simulink model "sampleModel111"  (Simulink 9.1)
settings: Solver=VariableStepAuto  StartTime=0.0  StopTime=10.0  RelTol=1e-3
undefined symbols (not defined in the file): DiscIntNeverNeededParam, Newton, Raphson
libraries: simulink x41
(part 1 of 2)
settings Model: Creator=DELL  LastModifiedBy=DELL
settings DataIOCC: SaveFormat=Dataset
settings OptimizationCC: LifeSpan=auto
settings DebuggingCC: UnderspecifiedInitializationDetection=Simplified  MergeDetectMultiDrivingBlocksExec=error  SFUnexpectedBacktrackingDiag=error  SFNoUnconditionalDefaultTransitionDiag=error  SFExecutionAtInitializationDiag=warning
settings HardwareCC: ProdBitPerPointer=64  ProdBitPerSizeT=64  ProdBitPerPtrDiffT=64  ProdLargestAtomicFloat=Float  ProdIntDivRoundTo=Zero  ProdEndianess=LittleEndian  ProdWordSize=64  ProdHWDeviceType=Intel->x86-64 (Windows64)
settings ModelReferenceCC: PropagateSignalLabelsOutOfModel=on
settings CodeAppCC: StateflowObjectComments=off
settings GRTTargetCC: TargetLangStandard=C99 (ISO)  CombineOutputUpdateFcns=on  GRTInterface=off
settings ConfigComp: CovMetricSettings=dwe  CovHtmlReporting=off  CovSaveCumulativeToWorkspaceVar=off  CovSaveSingleToWorkspaceVar=off  CovExternalEMLEnable=on

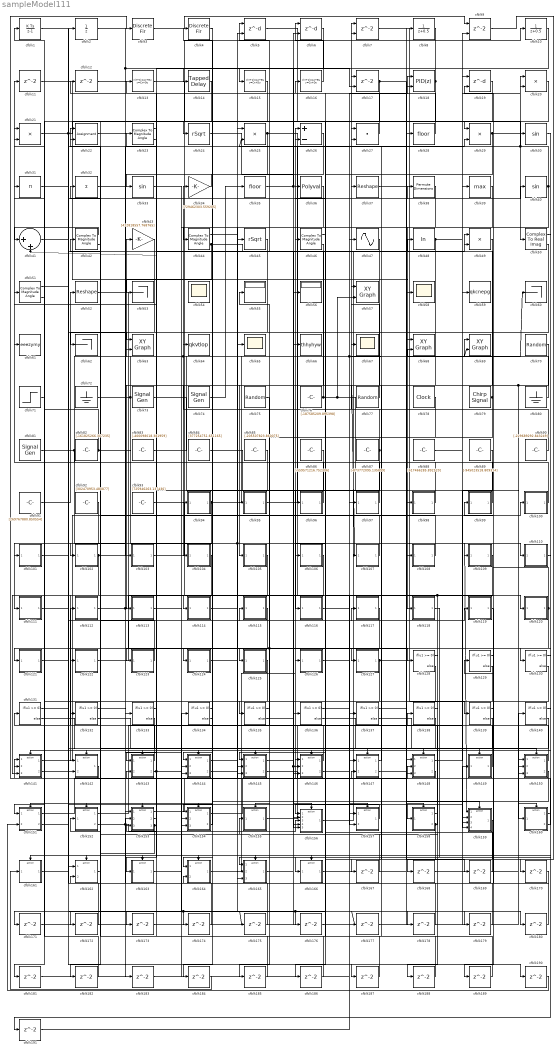
== system sampleModel111 ==
  cfblk1 : DiscreteIntegrator  ICPrevOutput=DiscIntNeverNeededParam  ICPrevScaledInput=DiscIntNeverNeededParam
  cfblk10 : DiscreteTransferFcn  SampleTime=1
  cfblk100 : Subsystem
  cfblk101 : Subsystem
  cfblk102 : Subsystem
  cfblk103 : Subsystem
  cfblk104 : Subsystem
  cfblk105 : Subsystem
  cfblk106 : Subsystem
  cfblk107 : Subsystem
  cfblk108 : Subsystem
  cfblk109 : Subsystem
  cfblk{11..12,167..191} (27 alike) : Delay  SampleTime=1
  cfblk110 : Subsystem
  cfblk111 : Subsystem
  cfblk112 : Subsystem
  cfblk113 : Subsystem
  cfblk114 : Subsystem
  cfblk115 : Subsystem
  cfblk116 : Subsystem
  cfblk117 : Subsystem
  cfblk118 : Subsystem
  cfblk119 : Subsystem
  cfblk120 : Subsystem
  cfblk121 : Subsystem
  cfblk122 : Subsystem
  cfblk123 : Subsystem
  cfblk124 : Subsystem
  cfblk125 : Subsystem
  cfblk126 : Subsystem
  cfblk127 : Subsystem
  cfblk{128..140} (13 alike) : If  IfExpression=u1 >= 0  SampleTime=1
  cfblk13 : DiscreteStateSpace
  cfblk14 : simulink/Discrete/Tapped Delay  vinit=0.0  samptime=-1  NumDelays=1  DelayOrder=Oldest  includeCurrent=off
  cfblk141 : Subsystem  TreatAsAtomicUnit=on
  cfblk142 : Subsystem  TreatAsAtomicUnit=on
  cfblk143 : Subsystem  TreatAsAtomicUnit=on
  cfblk144 : Subsystem  TreatAsAtomicUnit=on
  cfblk145 : Subsystem  TreatAsAtomicUnit=on
  cfblk146 : Subsystem  TreatAsAtomicUnit=on
  cfblk147 : Subsystem  TreatAsAtomicUnit=on
  cfblk148 : Subsystem  TreatAsAtomicUnit=on
  cfblk149 : Subsystem  TreatAsAtomicUnit=on
  cfblk15 : DiscreteStateSpace
  cfblk150 : Subsystem  TreatAsAtomicUnit=on
  cfblk151 : Subsystem  TreatAsAtomicUnit=on
  cfblk152 : Subsystem  TreatAsAtomicUnit=on
  cfblk153 : Subsystem  TreatAsAtomicUnit=on
  cfblk154 : Subsystem  TreatAsAtomicUnit=on
  cfblk155 : Subsystem  TreatAsAtomicUnit=on
  cfblk156 : Subsystem  TreatAsAtomicUnit=on
  cfblk157 : Subsystem  TreatAsAtomicUnit=on
  cfblk158 : Subsystem  TreatAsAtomicUnit=on
  cfblk159 : Subsystem  TreatAsAtomicUnit=on
  cfblk16 : DiscreteStateSpace
  cfblk160 : Subsystem  TreatAsAtomicUnit=on
  cfblk161 : Subsystem  TreatAsAtomicUnit=on
  cfblk162 : Subsystem  TreatAsAtomicUnit=on
  cfblk163 : Subsystem  TreatAsAtomicUnit=on
  cfblk164 : Subsystem  TreatAsAtomicUnit=on
  cfblk165 : Subsystem  TreatAsAtomicUnit=on
  cfblk166 : Subsystem  TreatAsAtomicUnit=on
  cfblk17 : Delay  ShowEnablePort=on  SampleTime=1
      settings: InputPortMap=u0,e6
  cfblk18 : simulink/Continuous/PID Controller (2DOF)  Controller=PID  TimeDomain=Discrete-time  SampleTime=1  IntegratorMethod=Forward Euler  FilterMethod=Forward Euler  Form=Parallel  UseFilter=on  ControllerParametersSource=internal  P=1  I=1  D=0  N=100  b=1  c=1  InitialConditionSource=internal  InitialConditionForIntegrator=0  InitialConditionForFilter=0  ExternalReset=none  LimitOutput=off  UpperSaturationLimit=inf  LowerSaturationLimit=-inf  LinearizeAsGain=off  AntiWindupMode=none  Kb=1  TrackingMode=off  Kt=1  PParamMin=[]  PParamMax=[]  IParamMin=[]  IParamMax=[]  DParamMin=[]  DParamMax=[]  NParamMin=[]  NParamMax=[]  bParamMin=[]  bParamMax=[]  cParamMin=[]  cParamMax=[]  KbParamMin=[]  KbParamMax=[]  KtParamMin=[]  KtParamMax=[]  POutMin=[]  POutMax=[]  IOutMin=[]  IOutMax=[]  DOutMin=[]  DOutMax=[]  NOutMin=[]  NOutMax=[]  bOutMin=[]  bOutMax=[]  cOutMin=[]  cOutMax=[]  KbOutMin=[]  KbOutMax=[]  KtOutMin=[]  KtOutMax=[]  IntegratorOutMin=[]  IntegratorOutMax=[]  FilterOutMin=[]  FilterOutMax=[]  SumOutMin=[]  SumOutMax=[]  Sum1OutMin=[]  Sum1OutMax=[]  Sum2OutMin=[]  Sum2OutMax=[]  Sum3OutMin=[]  Sum3OutMax=[]  SumI1OutMin=[]  SumI1OutMax=[]  SumI2OutMin=[]  SumI2OutMax=[]  SumI3OutMin=[]  SumI3OutMax=[]  SumDOutMin=[]  SumDOutMax=[]  SaturationOutMin=[]  SaturationOutMax=[]  IntegratorContinuousStateAttributes=''  IntegratorStateMustResolveToSignalObject=off  IntegratorRTWStateStorageClass=Auto  FilterContinuousStateAttributes=''  FilterStateMustResolveToSignalObject=off  FilterRTWStateStorageClass=Auto  DifferentiatorICPrevScaledInput=0  DifferentiatorOutMin=[]  DifferentiatorOutMax=[]  FilterDiffOutCoefMin=[]  FilterDiffOutCoefMax=[]  SumDenOutMin=[]  SumDenOutMax=[]  SumNumOutMin=[]  SumNumOutMax=[]  ReciprocalOutMin=[]  ReciprocalOutMax=[]  DivideOutMin=[]  DivideOutMax=[]  TunerSelectOption=Transfer Function Based (PID Tuner App)
  cfblk19 : Delay  DelayLengthSource=Input port  SampleTime=1
      settings: InputPortMap=u0,p1
  cfblk2 : UnitDelay
  cfblk20 : Product  Inputs=**
  cfblk21 : Product  Inputs=**
  cfblk22 : Assignment  DiagnosticForDimensions=Warning  IndexOptions=Index vector (dialog)  Indices=1  OutputSizes=1
  cfblk{23,42,44,46,51} (5 alike) : ComplexToMagnitudeAngle
  cfblk24 : Sqrt  Operator=rSqrt  AlgorithmType=Newton-Raphson  SaturateOnIntegerOverflow=on
  cfblk25 : Product
  cfblk26 : Sum  Inputs=+-
  cfblk27 : DotProduct  InputSameDT=on  OutDataTypeStr=Inherit: Inherit via internal rule
  cfblk28 : Rounding
  cfblk29 : Product  Inputs=**
  cfblk3 : DiscreteFir  SampleTime=1
  cfblk30 : Trigonometry
  cfblk31 : Product  Inputs=*
  cfblk32 : Sum  Inputs=+
  cfblk33 : Trigonometry
  cfblk34 : Gain  Gain=[729462303.559205]
  cfblk35 : Rounding
  cfblk36 : Polyval  Coefs=[ +2.081618890e-019, -1.441693666e-014, +4.719686976e-010, -8.536869453e-006, +1.621573104e-001, -8.087801117e+001 ]
  cfblk37 : Reshape
  cfblk38 : PermuteDimensions
  cfblk39 : MinMax  Function=max
  cfblk4 : DiscreteFir  SampleTime=1
  cfblk40 : Trigonometry
  cfblk41 : Sum  Inputs=|++
  cfblk43 : Gain  Gain=[412818557.768765]
  cfblk45 : Sqrt  Operator=rSqrt  AlgorithmType=Newton-Raphson  SaturateOnIntegerOverflow=on
  cfblk47 : Sin  TimeSource=Use external signal  SampleTime=0
  cfblk48 : Math  Operator=log  SaturateOnIntegerOverflow=on
  cfblk49 : Product
  cfblk5 : Delay  DelayLengthSource=Input port  SampleTime=1
      settings: InputPortMap=u0,p1
  cfblk50 : ComplexToRealImag
  cfblk52 : Reshape
  cfblk53 : Terminator
  cfblk{54,58,65,67} (4 alike) : Scope
      cfblk54 settings: Floating=on
  cfblk55 : Display
  cfblk56 : Display
  cfblk{57,63,68..69} (4 alike) : simulink/Sinks/XY Graph  xmin=-1  xmax=1  ymin=-1  ymax=1  st=-1
  cfblk59 : ToWorkspace  VariableName=qkcnepg  SaveFormat=Timeseries  SampleTime=-1
  cfblk6 : Delay  DelayLengthSource=Input port  SampleTime=1
      settings: InputPortMap=u0,p1
  cfblk60 : Terminator
  cfblk61 : ToWorkspace  VariableName=eeezymy  SaveFormat=Timeseries  SampleTime=-1
  cfblk62 : Terminator
  cfblk64 : ToWorkspace  VariableName=qkvtlop  SaveFormat=Timeseries  SampleTime=-1
  cfblk66 : ToWorkspace  VariableName=thhyhyw  SaveFormat=Timeseries  SampleTime=-1
  cfblk7 : Delay  ShowEnablePort=on  SampleTime=1
      settings: InputPortMap=u0,e6
  cfblk70 : RandomNumber  Mean=[-93187.376150]  Variance=[1459.067159]  Seed=[649544594.000000]  SampleTime=0.1
  cfblk71 : Step  Time=[20.000000]  Before=[-473754726.003324]  After=[611327295.149890]  SampleTime=0
  cfblk72 : Ground
  cfblk73 : SignalGenerator  WaveForm=square  Amplitude=[306363798.887953]
  cfblk74 : SignalGenerator  WaveForm=square  Amplitude=[94323336.966715]
  cfblk75 : RandomNumber  Mean=[-15248.816156]  Variance=[85638.241331]  Seed=[321907178.000000]  SampleTime=0.1
  cfblk76 : Constant  Value=[-187585209.895398]  SampleTime=1
  cfblk77 : RandomNumber  Mean=[-59356.286087]  Variance=[90170.885384]  Seed=[654352613.000000]  SampleTime=0.1
  cfblk78 : DigitalClock
  cfblk79 : simulink/Sources/Chirp Signal  f1=[-120890436.083449]  T=[764356880.898604]  f2=[390283398.799809]
  cfblk8 : DiscreteTransferFcn  SampleTime=1
  cfblk80 : Ground
  cfblk81 : SignalGenerator  WaveForm=square  Amplitude=[-879054946.376527]  Units=rad/sec
  cfblk82 : Constant  Value=[-161825266.307235]  SampleTime=1
  cfblk83 : Constant  Value=[-400098018.381959]  SampleTime=1
  cfblk84 : Constant  Value=[377254751.651165]  SampleTime=1
  cfblk85 : Constant  Value=[-205507823.860075]  SampleTime=1
  cfblk86 : Constant  Value=[-559571216.752306]  SampleTime=1
  cfblk87 : Constant  Value=[-873772095.135899]  SampleTime=1
  cfblk88 : Constant  Value=[617466285.892520]  SampleTime=1
  cfblk89 : Constant  Value=[-945023518.809314]  SampleTime=1
  cfblk9 : Delay  ShowEnablePort=on  SampleTime=1
      settings: InputPortMap=u0,e6
  cfblk90 : Constant  Value=[-229689292.843249]  SampleTime=1
  cfblk91 : Constant  Value=[269767880.850554]  SampleTime=1
  cfblk92 : Constant  Value=[302470953.480877]  SampleTime=1
  cfblk93 : Constant  Value=[725946263.137430]  SampleTime=1
  cfblk94 : Subsystem
  cfblk95 : Subsystem
  cfblk96 : Subsystem
  cfblk97 : Subsystem
  cfblk98 : Subsystem
  cfblk99 : Subsystem
  wires:
  cfblk82/1 -> cfblk159/1(cfblk1), cfblk145/3(cfblk13), cfblk1/1
  cfblk154/1(cfblk2) -> cfblk26/1
  cfblk158/1(cfblk2) -> cfblk43/1
  cfblk118/1(cfblk2) -> cfblk166/1(cfblk1)
  cfblk103/1(cfblk2) -> cfblk10/1
  cfblk3/1 -> cfblk9/1
  cfblk17/1 -> cfblk96/1(cfblk1), cfblk169/1
  cfblk156/1(cfblk2) -> cfblk49/1
  cfblk141/1(cfblk2) -> cfblk100/1(cfblk1)
  cfblk7/1 -> cfblk109/1(cfblk1)
  cfblk74/1 -> cfblk35/1
  cfblk37/1 -> cfblk139/1
  cfblk6/1 -> cfblk163/1(cfblk1)
  cfblk70/1 -> cfblk107/1(cfblk1), cfblk150/3(cfblk7)
  cfblk25/1 -> cfblk120/1(cfblk1), cfblk123/1(cfblk1)
  cfblk95/1(cfblk2) -> cfblk7/1
  cfblk87/1 -> cfblk7/2, cfblk143/1(cfblk1)
  cfblk77/1 -> cfblk57/1
  cfblk164/1(cfblk2) -> cfblk126/1(cfblk1)
  cfblk99/1(cfblk2) -> cfblk11/1
  cfblk79/1 -> cfblk146/2(cfblk13), cfblk156/5(cfblk16), cfblk5/1
  cfblk14/1 -> cfblk24/1
  cfblk34/1 -> cfblk33/1
  cfblk90/1 -> cfblk34/1
  cfblk39/1 -> cfblk118/1(cfblk1)
  cfblk32/1 -> cfblk127/1(cfblk1)
  cfblk2/1 -> cfblk133/1, cfblk17/2
  cfblk122/1(cfblk2) -> cfblk117/1(cfblk1)
  cfblk52/1 -> cfblk124/1(cfblk1)
  cfblk91/1 -> cfblk52/1
  cfblk46/1 -> cfblk145/1(cfblk1)
  cfblk33/1 -> cfblk58/1
  cfblk26/1 -> cfblk144/1(cfblk1)
  cfblk92/1 -> cfblk111/1(cfblk1)
  cfblk153/1(cfblk2) -> cfblk65/1
  cfblk48/1 -> cfblk20/1, cfblk95/1(cfblk1)
  cfblk142/1(cfblk2) -> cfblk3/1
  cfblk105/1(cfblk2) -> cfblk164/1(cfblk1)
  cfblk145/1(cfblk2) -> cfblk56/1
  cfblk150/1(cfblk2) -> cfblk99/1(cfblk1)
  cfblk102/1(cfblk2) -> cfblk142/1(cfblk1), cfblk27/2
  cfblk141/2(cfblk9) -> cfblk174/1, cfblk175/1
  cfblk147/1(cfblk2) -> cfblk67/1
  cfblk81/1 -> cfblk45/1, cfblk153/1(cfblk1)
  cfblk11/1 -> cfblk108/1(cfblk1)
  cfblk85/1 -> cfblk105/1(cfblk1)
  cfblk83/1 -> cfblk8/1
  cfblk112/1(cfblk2) -> cfblk114/1(cfblk1), cfblk178/1
  cfblk162/1(cfblk2) -> cfblk42/1
  cfblk96/1(cfblk2) -> cfblk13/1
  cfblk50/1 -> cfblk165/1(cfblk1)
  cfblk94/1(cfblk2) -> cfblk9/2, cfblk102/1(cfblk1)
  cfblk109/1(cfblk2) -> cfblk186/1, cfblk188/1
  cfblk113/1(cfblk2) -> cfblk158/1(cfblk1)
  cfblk158/2(cfblk17) -> cfblk138/1, cfblk171/1
  cfblk84/1 -> cfblk98/1(cfblk1)
  cfblk86/1 -> cfblk116/1(cfblk1)
  cfblk13/1 -> cfblk68/1
  cfblk24/1 -> cfblk66/1
  cfblk47/1 -> cfblk113/1(cfblk1)
  cfblk123/1(cfblk2) -> cfblk32/1
  cfblk151/1(cfblk2) -> cfblk25/1
  cfblk151/2(cfblk16) -> cfblk115/1(cfblk1)
  cfblk5/1 -> cfblk50/1
  cfblk97/1(cfblk2) -> cfblk61/1
  cfblk98/1(cfblk2) -> cfblk36/1
  cfblk93/1 -> cfblk157/1(cfblk1)
  cfblk127/1(cfblk2) -> cfblk165/2(cfblk10), cfblk69/1
  cfblk89/1 -> cfblk159/2(cfblk14)
  cfblk149/1(cfblk2) -> cfblk55/1
  cfblk15/1 -> cfblk44/1
  cfblk44/1 -> cfblk110/1(cfblk1)
  cfblk88/1 -> cfblk19/1
  cfblk45/1 -> cfblk62/1
  cfblk16/1 -> cfblk6/1
  cfblk78/1 -> cfblk125/1(cfblk1)
  cfblk23/1 -> cfblk121/1(cfblk1)
  cfblk116/1(cfblk2) -> cfblk18/1, cfblk69/2
  cfblk31/1 -> cfblk63/1
  cfblk35/1 -> cfblk6/2, cfblk128/1
  cfblk163/1(cfblk2) -> cfblk148/2(cfblk12)
  cfblk120/1(cfblk2) -> cfblk154/1(cfblk1), cfblk19/2
  cfblk76/1 -> cfblk57/2, cfblk150/2(cfblk6), cfblk23/1
  cfblk165/1(cfblk2) -> cfblk49/2
  cfblk155/1(cfblk2) -> cfblk59/1
  cfblk40/1 -> cfblk20/2, cfblk25/2, cfblk146/3(cfblk14)
  cfblk73/1 -> cfblk160/1(cfblk1)
  cfblk143/1(cfblk2) -> cfblk112/1(cfblk1)
  cfblk125/1(cfblk2) -> cfblk151/1(cfblk1)
  cfblk166/1(cfblk2) -> cfblk28/1
  cfblk154/2(cfblk10) -> cfblk12/1
  cfblk147/2(cfblk17) -> cfblk18/2
  cfblk111/1(cfblk2) -> cfblk40/1
  cfblk42/1 -> cfblk41/1
  cfblk23/2 -> cfblk103/1(cfblk1)
  cfblk8/1 -> cfblk15/1
  cfblk72/1 -> cfblk60/1, cfblk64/1, cfblk159/3(cfblk15)
  cfblk144/1(cfblk2) -> cfblk37/1
  cfblk21/1 -> cfblk29/1, cfblk29/2
  cfblk108/1(cfblk2) -> cfblk22/1
  cfblk148/1(cfblk2) -> cfblk39/1
  cfblk121/1(cfblk2) -> cfblk2/1
  cfblk38/1 -> cfblk154/2(cfblk8)
  cfblk143/2(cfblk10) -> cfblk41/2, cfblk179/1
  cfblk41/1 -> cfblk159/4(cfblk16)
  cfblk106/1(cfblk2) -> cfblk142/2(cfblk10)
  cfblk50/2 -> cfblk165/3(cfblk11)
  cfblk44/2 -> cfblk46/1, cfblk53/1
  cfblk152/1(cfblk2) -> cfblk97/1(cfblk1)
  cfblk18/1 -> cfblk14/1, cfblk156/4(cfblk15)
  cfblk107/1(cfblk2) -> cfblk16/1
  cfblk19/1 -> cfblk101/1(cfblk1)
  cfblk42/2 -> cfblk122/1(cfblk1)
  cfblk1/1 -> cfblk157/2(cfblk9)
  cfblk29/1 -> cfblk106/1(cfblk1), cfblk30/1
  cfblk157/1(cfblk2) -> cfblk156/1(cfblk1)
  cfblk71/1 -> cfblk31/1
  cfblk152/2(cfblk10) -> cfblk156/3(cfblk14), cfblk187/1
  cfblk46/2 -> cfblk104/1(cfblk1)
  cfblk115/1(cfblk2) -> cfblk154/3(cfblk9)
  cfblk10/1 -> cfblk156/2(cfblk13)
  cfblk145/2(cfblk14) -> cfblk148/3(cfblk13)
  cfblk161/1(cfblk2) -> cfblk48/1
  cfblk43/1 -> cfblk63/2
  cfblk28/1 -> cfblk4/1
  cfblk153/2(cfblk12) -> cfblk141/1(cfblk1)
  cfblk80/1 -> cfblk68/2
  cfblk114/1(cfblk2) -> cfblk176/1, cfblk177/1
  cfblk153/3(cfblk13) -> cfblk51/1, cfblk182/1
  cfblk36/1 -> cfblk145/2(cfblk12)
  cfblk100/1(cfblk2) -> cfblk27/1
  cfblk117/1(cfblk2) -> cfblk132/1, cfblk185/1
  cfblk110/1(cfblk2) -> cfblk130/1
  cfblk12/1 -> cfblk144/3(cfblk12)
  cfblk27/1 -> cfblk17/1
  cfblk160/2(cfblk12) -> cfblk141/2(cfblk7)
  cfblk4/1 -> cfblk94/1(cfblk1)
  cfblk126/1(cfblk2) -> cfblk47/1
  cfblk124/1(cfblk2) -> cfblk38/1
  cfblk146/1(cfblk2) -> cfblk21/1
  cfblk148/2(cfblk14) -> cfblk146/1(cfblk1)
  cfblk104/1(cfblk2) -> cfblk141/3(cfblk8)
  cfblk146/2(cfblk15) -> cfblk119/1(cfblk1)
  cfblk75/1 -> cfblk135/1
  cfblk144/2(cfblk13) -> cfblk5/2
  cfblk128/1 -> cfblk141/Action
  cfblk128/2 -> cfblk142/Action
  cfblk129/1 -> cfblk143/Action
  cfblk129/2 -> cfblk144/Action
  cfblk130/1 -> cfblk145/Action
  cfblk130/2 -> cfblk146/Action
  cfblk131/1 -> cfblk147/Action
  cfblk131/2 -> cfblk148/Action
  cfblk132/1 -> cfblk149/Action
  cfblk132/2 -> cfblk150/Action
  cfblk133/1 -> cfblk151/Action
  cfblk133/2 -> cfblk152/Action
  cfblk134/1 -> cfblk153/Action
  cfblk134/2 -> cfblk154/Action
  cfblk135/1 -> cfblk155/Action
  cfblk135/2 -> cfblk156/Action
  cfblk136/1 -> cfblk157/Action
  cfblk136/2 -> cfblk158/Action
  cfblk137/1 -> cfblk159/Action
  cfblk137/2 -> cfblk160/Action
  cfblk138/1 -> cfblk161/Action
  cfblk138/2 -> cfblk162/Action
  cfblk139/1 -> cfblk163/Action
  cfblk139/2 -> cfblk164/Action
  cfblk140/1 -> cfblk165/Action
  cfblk140/2 -> cfblk166/Action
  cfblk49/1 -> cfblk167/1
  cfblk167/1 -> cfblk155/1(cfblk1)
  cfblk9/1 -> cfblk168/1
  cfblk168/1 -> cfblk140/1
  cfblk169/1 -> cfblk131/1
  cfblk30/1 -> cfblk170/1
  cfblk170/1 -> cfblk164/2(cfblk15)
  cfblk171/1 -> cfblk136/1
  cfblk20/1 -> cfblk172/1
  cfblk172/1 -> cfblk162/2(cfblk7)
  cfblk159/1(cfblk2) -> cfblk173/1
  cfblk173/1 -> cfblk148/1(cfblk1)
  cfblk174/1 -> cfblk162/1(cfblk1)
  cfblk175/1 -> cfblk22/2
  cfblk176/1 -> cfblk150/1(cfblk1)
  cfblk177/1 -> cfblk149/1(cfblk1)
  cfblk178/1 -> cfblk143/2(cfblk9)
  cfblk179/1 -> cfblk153/2(cfblk10)
  cfblk51/1 -> cfblk180/1
  cfblk180/1 -> cfblk129/1
  cfblk51/2 -> cfblk181/1
  cfblk181/1 -> cfblk147/1(cfblk1)
  cfblk182/1 -> cfblk21/2
  cfblk22/1 -> cfblk183/1
  cfblk183/1 -> cfblk134/1
  cfblk150/2(cfblk8) -> cfblk184/1
  cfblk184/1 -> cfblk161/1(cfblk1)
  cfblk185/1 -> cfblk153/3(cfblk11)
  cfblk186/1 -> cfblk152/1(cfblk1)
  cfblk187/1 -> cfblk144/2(cfblk11)
  cfblk188/1 -> cfblk147/2(cfblk16)
  cfblk119/1(cfblk2) -> cfblk189/1
  cfblk189/1 -> cfblk26/2
  cfblk101/1(cfblk2) -> cfblk190/1
  cfblk190/1 -> cfblk151/2(cfblk15)
  cfblk160/1(cfblk2) -> cfblk191/1
  cfblk191/1 -> cfblk137/1

== system sampleModel111/cfblk100 ==
  cfblk1 : Inport
  cfblk2 : Outport
  wires:
  cfblk1/1 -> cfblk2/1

== system sampleModel111/cfblk101 ==
  cfblk1 : Inport
  cfblk2 : Outport
  wires:
  cfblk1/1 -> cfblk2/1

== system sampleModel111/cfblk102 ==
  cfblk1 : Inport
  cfblk2 : Outport
  wires:
  cfblk1/1 -> cfblk2/1

== system sampleModel111/cfblk103 ==
  cfblk1 : Inport
  cfblk2 : Outport
  wires:
  cfblk1/1 -> cfblk2/1

== system sampleModel111/cfblk104 ==
  cfblk1 : Inport
  cfblk2 : Outport
  wires:
  cfblk1/1 -> cfblk2/1

== system sampleModel111/cfblk105 ==
  cfblk1 : Inport
  cfblk2 : Outport
  wires:
  cfblk1/1 -> cfblk2/1

== system sampleModel111/cfblk106 ==
  cfblk1 : Inport
  cfblk2 : Outport
  wires:
  cfblk1/1 -> cfblk2/1

== system sampleModel111/cfblk107 ==
  cfblk1 : Inport
  cfblk2 : Outport
  wires:
  cfblk1/1 -> cfblk2/1

== system sampleModel111/cfblk108 ==
  cfblk1 : Inport
  cfblk2 : Outport
  wires:
  cfblk1/1 -> cfblk2/1

== system sampleModel111/cfblk109 ==
  cfblk1 : Inport
  cfblk2 : Outport
  wires:
  cfblk1/1 -> cfblk2/1

== system sampleModel111/cfblk110 ==
  cfblk1 : Inport
  cfblk2 : Outport
  wires:
  cfblk1/1 -> cfblk2/1

== system sampleModel111/cfblk111 ==
  cfblk1 : Inport
  cfblk2 : Outport
  wires:
  cfblk1/1 -> cfblk2/1

== system sampleModel111/cfblk112 ==
  cfblk1 : Inport
  cfblk2 : Outport
  wires:
  cfblk1/1 -> cfblk2/1

== system sampleModel111/cfblk113 ==
  cfblk1 : Inport
  cfblk2 : Outport
  wires:
  cfblk1/1 -> cfblk2/1

== system sampleModel111/cfblk114 ==
  cfblk1 : Inport
  cfblk2 : Outport
  wires:
  cfblk1/1 -> cfblk2/1

== system sampleModel111/cfblk115 ==
  cfblk1 : Inport
  cfblk2 : Outport
  wires:
  cfblk1/1 -> cfblk2/1

== system sampleModel111/cfblk116 ==
  cfblk1 : Inport
  cfblk2 : Outport
  wires:
  cfblk1/1 -> cfblk2/1

== system sampleModel111/cfblk117 ==
  cfblk1 : Inport
  cfblk2 : Outport
  wires:
  cfblk1/1 -> cfblk2/1

== system sampleModel111/cfblk118 ==
  cfblk1 : Inport
  cfblk2 : Outport
  wires:
  cfblk1/1 -> cfblk2/1

== system sampleModel111/cfblk119 ==
  cfblk1 : Inport
  cfblk2 : Outport
  wires:
  cfblk1/1 -> cfblk2/1

== system sampleModel111/cfblk120 ==
  cfblk1 : Inport
  cfblk2 : Outport
  wires:
  cfblk1/1 -> cfblk2/1

== system sampleModel111/cfblk121 ==
  cfblk1 : Inport
  cfblk2 : Outport
  wires:
  cfblk1/1 -> cfblk2/1

== system sampleModel111/cfblk122 ==
  cfblk1 : Inport
  cfblk2 : Outport
  wires:
  cfblk1/1 -> cfblk2/1

== system sampleModel111/cfblk123 ==
  cfblk1 : Inport
  cfblk2 : Outport
  wires:
  cfblk1/1 -> cfblk2/1

== system sampleModel111/cfblk124 ==
  cfblk1 : Inport
  cfblk2 : Outport
  wires:
  cfblk1/1 -> cfblk2/1

== system sampleModel111/cfblk125 ==
  cfblk1 : Inport
  cfblk2 : Outport
  wires:
  cfblk1/1 -> cfblk2/1

== system sampleModel111/cfblk126 ==
  cfblk1 : Inport
  cfblk2 : Outport
  wires:
  cfblk1/1 -> cfblk2/1

== system sampleModel111/cfblk127 ==
  cfblk1 : Inport
  cfblk2 : Outport
  wires:
  cfblk1/1 -> cfblk2/1

== system sampleModel111/cfblk141 ==
  cfblk1 : Inport
  cfblk7 : Inport  Port=2
  cfblk8 : Inport  Port=3
  Action Port : ActionPort  ActionType=then
  cfblk3 : simulink/Discrete/Transfer Fcn Real Zero  ZeroZ=0.75  ICPrevInput=0.0  DoSatur=off
      settings: SourceProductName=Simulink  SourceProductBaseCode=SL
  cfblk4 : Constant  Value=[558224029.714252]  SampleTime=1
  cfblk5 : Constant  Value=[-623702994.470588]  SampleTime=1
  cfblk6 : Subsystem
  cfblk2 : Outport
  cfblk9 : Outport  Port=2
  wires:
  cfblk4/1 -> cfblk6/1(cfblk1)
  cfblk5/1 -> cfblk2/1
  cfblk7/1 -> cfblk9/1
  cfblk8/1 -> cfblk3/1

== system sampleModel111/cfblk142 ==
  cfblk1 : Inport
  cfblk10 : Inport  Port=2
  Action Port : ActionPort  ActionType=else
  cfblk11 : Delay
  cfblk3 : simulink/Discrete/Tapped Delay  vinit=0.0  samptime=-1  NumDelays=1  DelayOrder=Oldest  includeCurrent=off
  cfblk4 : simulink/Math Operations/MinMax Running Resettable  Function=min  vinit=0.0
  cfblk5 : ComplexToMagnitudeAngle
  cfblk6 : Subsystem
  cfblk7 : Subsystem
  cfblk8 : Subsystem
  cfblk9 : Subsystem
  cfblk2 : Outport
  wires:
  cfblk6/1(cfblk2) -> cfblk7/1(cfblk1)
  cfblk7/1(cfblk2) -> cfblk4/1
  cfblk3/1 -> cfblk8/1(cfblk1)
  cfblk4/1 -> cfblk9/1(cfblk1)
  cfblk5/1 -> cfblk6/1(cfblk1)
  cfblk5/2 -> cfblk3/1
  cfblk10/1 -> cfblk5/1
  cfblk8/1(cfblk2) -> cfblk2/1
  cfblk9/1(cfblk2) -> cfblk11/1
  cfblk11/1 -> cfblk4/2

== system sampleModel111/cfblk143 ==
  cfblk1 : Inport
  cfblk9 : Inport  Port=2
  Action Port : ActionPort  ActionType=then
  cfblk11 : Subsystem  TreatAsAtomicUnit=on
  cfblk12 : Subsystem  TreatAsAtomicUnit=on
  cfblk13 : Delay
  cfblk3 : Bias  Bias=[170182456.722809]
  cfblk4 : Math  Operator=conj  SaturateOnIntegerOverflow=on
  cfblk5 : Subsystem
  cfblk6 : Subsystem
  cfblk7 : Subsystem
  cfblk8 : If  IfExpression=u1 >= 0  SampleTime=1
  cfblk2 : Outport
  cfblk10 : Outport  Port=2
  wires:
  cfblk6/1(cfblk2) -> cfblk4/1
  cfblk1/1 -> cfblk8/1, cfblk12/2(cfblk10)
  cfblk9/1 -> cfblk6/1(cfblk1), cfblk3/1, cfblk11/4(cfblk15)
  cfblk4/1 -> cfblk7/1(cfblk1)
  cfblk3/1 -> cfblk12/1(cfblk1)
  cfblk11/1(cfblk2) -> cfblk10/1
  cfblk11/2(cfblk16) -> cfblk5/1(cfblk1)
  cfblk7/1(cfblk2) -> cfblk2/1
  cfblk12/1(cfblk2) -> cfblk11/2(cfblk13)
  cfblk12/2(cfblk11) -> cfblk11/3(cfblk14)
  cfblk8/1 -> cfblk11/Action
  cfblk8/2 -> cfblk12/Action
  cfblk5/1(cfblk2) -> cfblk13/1
  cfblk13/1 -> cfblk11/1(cfblk1)

== system sampleModel111/cfblk144 ==
  cfblk1 : Inport
  cfblk11 : Inport  Port=2
  cfblk12 : Inport  Port=3
  Action Port : ActionPort  ActionType=else
  cfblk10 : Subsystem
  cfblk3 : DiscreteStateSpace  SampleTime=-1
  cfblk4 : Delay  DelayLengthSource=Input port
      settings: InputPortMap=u0,p1
  cfblk5 : Abs
  cfblk6 : simulink/Math Operations/Slider Gain  gain=1  low=0  high=2
  cfblk7 : Subsystem
  cfblk8 : Subsystem
  cfblk9 : Subsystem
  cfblk2 : Outport
  cfblk13 : Outport  Port=2
  wires:
  cfblk4/1 -> cfblk3/1
  cfblk9/1(cfblk2) -> cfblk8/1(cfblk1)
  cfblk6/1 -> cfblk9/1(cfblk1)
  cfblk8/1(cfblk2) -> cfblk13/1
  cfblk10/1(cfblk2) -> cfblk5/1
  cfblk3/1 -> cfblk7/1(cfblk1)
  cfblk5/1 -> cfblk6/1
  cfblk7/1(cfblk2) -> cfblk2/1
  cfblk1/1 -> cfblk4/1
  cfblk12/1 -> cfblk10/1(cfblk1)
  cfblk11/1 -> cfblk4/2

== system sampleModel111/cfblk145 ==
  cfblk1 : Inport
  cfblk12 : Inport  Port=2
  cfblk13 : Inport  Port=3
  Action Port : ActionPort  ActionType=then
  cfblk10 : Subsystem
  cfblk11 : Subsystem
  cfblk15 : Delay
  cfblk3 : simulink/Discrete/Transfer Fcn Lead or Lag  PoleZ=0.95  ZeroZ=0.75  ICPrevOutput=0.0  ICPrevInput=0.0  DoSatur=off
      settings: SourceProductName=Simulink  SourceProductBaseCode=SL
  cfblk4 : Product  Inputs=*
  cfblk5 : Gain  Gain=[598328257.890365]
  cfblk6 : Sum  Inputs=+
  cfblk7 : Trigonometry
  cfblk8 : Subsystem
  cfblk9 : Subsystem
  cfblk2 : Outport
  cfblk14 : Outport  Port=2
  wires:
  cfblk1/1 -> cfblk7/1
  cfblk13/1 -> cfblk10/1(cfblk1)
  cfblk7/1 -> cfblk6/1
  cfblk8/1(cfblk2) -> cfblk2/1
  cfblk5/1 -> cfblk9/1(cfblk1)
  cfblk3/1 -> cfblk4/1
  cfblk6/1 -> cfblk8/1(cfblk1)
  cfblk10/1(cfblk2) -> cfblk11/1(cfblk1)
  cfblk11/1(cfblk2) -> cfblk5/1
  cfblk9/1(cfblk2) -> cfblk14/1
  cfblk4/1 -> cfblk15/1
  cfblk15/1 -> cfblk3/1

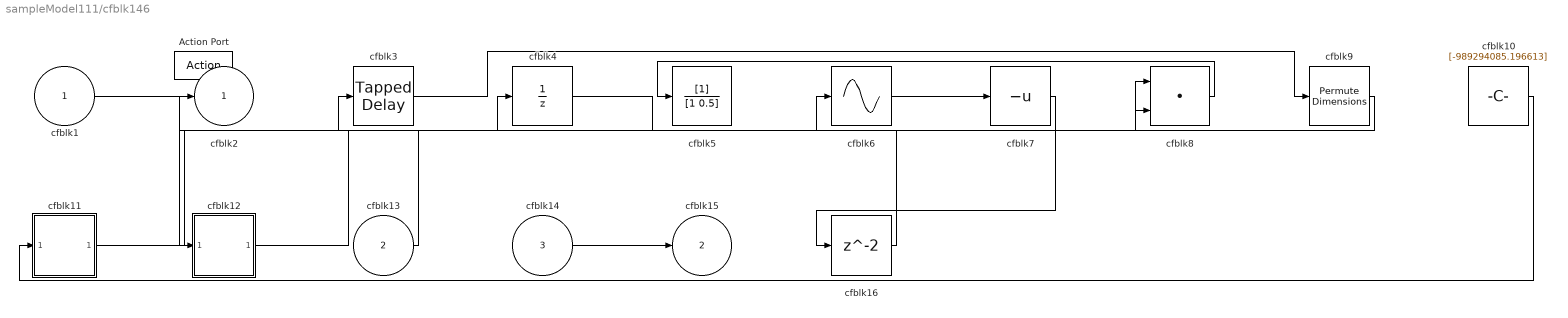
== system sampleModel111/cfblk146 ==
  cfblk1 : Inport
  cfblk13 : Inport  Port=2
  cfblk14 : Inport  Port=3
  Action Port : ActionPort  ActionType=else
  cfblk10 : Constant  Value=[-989294085.196613]  SampleTime=1
  cfblk11 : Subsystem
  cfblk12 : Subsystem
  cfblk16 : Delay
  cfblk3 : simulink/Discrete/Tapped Delay  vinit=0.0  samptime=-1  NumDelays=1  DelayOrder=Oldest  includeCurrent=off
  cfblk4 : UnitDelay  SampleTime=-1
  cfblk5 : DiscreteFilter
  cfblk6 : Sin  TimeSource=Use external signal  SampleTime=0
  cfblk7 : UnaryMinus
  cfblk8 : DotProduct  InputSameDT=on  OutDataTypeStr=Inherit: Inherit via internal rule
  cfblk9 : PermuteDimensions
  cfblk2 : Outport
  cfblk15 : Outport  Port=2
  wires:
  cfblk11/1(cfblk2) -> cfblk3/1
  cfblk6/1 -> cfblk7/1
  cfblk8/1 -> cfblk5/1
  cfblk1/1 -> cfblk12/1(cfblk1)
  cfblk14/1 -> cfblk15/1
  cfblk13/1 -> cfblk2/1
  cfblk9/1 -> cfblk4/1
  cfblk12/1(cfblk2) -> cfblk8/1
  cfblk10/1 -> cfblk11/1(cfblk1)
  cfblk4/1 -> cfblk8/2
  cfblk3/1 -> cfblk9/1
  cfblk7/1 -> cfblk16/1
  cfblk16/1 -> cfblk6/1

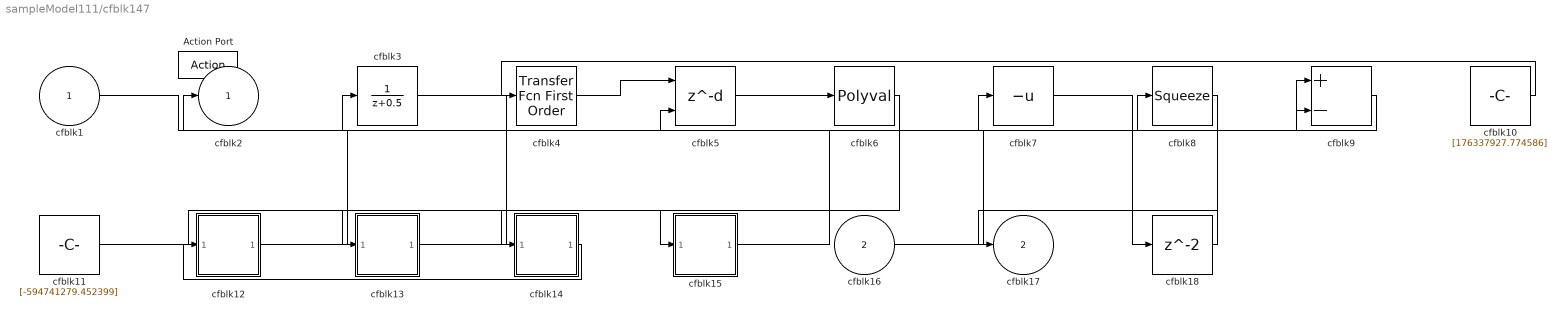
== system sampleModel111/cfblk147 ==
  cfblk1 : Inport
  cfblk16 : Inport  Port=2
  Action Port : ActionPort  ActionType=then
  cfblk10 : Constant  Value=[176337927.774586]  SampleTime=1
  cfblk11 : Constant  Value=[-594741279.452399]  SampleTime=1
  cfblk12 : Subsystem
  cfblk13 : Subsystem
  cfblk14 : Subsystem
  cfblk15 : Subsystem
  cfblk18 : Delay
  cfblk3 : DiscreteTransferFcn
  cfblk4 : simulink/Discrete/Transfer Fcn First Order  PoleZ=0.95  ICPrevOutput=0.0  DoSatur=off
      settings: SourceProductName=Simulink
  cfblk5 : Delay  DelayLengthSource=Input port
      settings: InputPortMap=u0,p1
  cfblk6 : Polyval  Coefs=[ +2.081618890e-019, -1.441693666e-014, +4.719686976e-010, -8.536869453e-006, +1.621573104e-001, -8.087801117e+001 ]
  cfblk7 : UnaryMinus
  cfblk8 : Squeeze
  cfblk9 : Sum  Inputs=+-
  cfblk2 : Outport
  cfblk17 : Outport  Port=2
  wires:
  cfblk9/1 -> cfblk2/1
  cfblk5/1 -> cfblk6/1
  cfblk4/1 -> cfblk5/1
  cfblk16/1 -> cfblk9/1
  cfblk13/1(cfblk2) -> cfblk8/1
  cfblk3/1 -> cfblk15/1(cfblk1)
  cfblk10/1 -> cfblk4/1
  cfblk11/1 -> cfblk14/1(cfblk1)
  cfblk15/1(cfblk2) -> cfblk7/1
  cfblk12/1(cfblk2) -> cfblk9/2
  cfblk8/1 -> cfblk17/1
  cfblk6/1 -> cfblk13/1(cfblk1)
  cfblk1/1 -> cfblk5/2
  cfblk14/1(cfblk2) -> cfblk12/1(cfblk1)
  cfblk7/1 -> cfblk18/1
  cfblk18/1 -> cfblk3/1

== system sampleModel111/cfblk148 ==
  cfblk1 : Inport
  cfblk12 : Inport  Port=2
  cfblk13 : Inport  Port=3
  Action Port : ActionPort  ActionType=else
  cfblk10 : Subsystem
  cfblk11 : Subsystem
  cfblk15 : Delay
  cfblk3 : simulink/Discrete/Transfer Fcn First Order  PoleZ=0.95  ICPrevOutput=0.0  DoSatur=off
      settings: SourceProductName=Simulink
  cfblk4 : simulink/Discrete/Transfer Fcn Lead or Lag  PoleZ=0.95  ZeroZ=0.75  ICPrevOutput=0.0  ICPrevInput=0.0  DoSatur=off
      settings: SourceProductName=Simulink  SourceProductBaseCode=SL
  cfblk5 : Sum  Inputs=+-
  cfblk6 : simulink/Math Operations/MinMax Running Resettable  Function=min  vinit=0.0
  cfblk7 : UnaryMinus
  cfblk8 : Rounding
  cfblk9 : Math  Operator=transpose  SaturateOnIntegerOverflow=on
  cfblk2 : Outport
  cfblk14 : Outport  Port=2
  wires:
  cfblk12/1 -> cfblk10/1(cfblk1)
  cfblk13/1 -> cfblk7/1
  cfblk6/1 -> cfblk2/1
  cfblk1/1 -> cfblk11/1(cfblk1)
  cfblk4/1 -> cfblk5/1
  cfblk7/1 -> cfblk5/2, cfblk9/1
  cfblk10/1(cfblk2) -> cfblk3/1
  cfblk11/1(cfblk2) -> cfblk6/1
  cfblk9/1 -> cfblk14/1
  cfblk3/1 -> cfblk8/1
  cfblk8/1 -> cfblk6/2
  cfblk5/1 -> cfblk15/1
  cfblk15/1 -> cfblk4/1

== system sampleModel111/cfblk149 ==
  cfblk1 : Inport
  Action Port : ActionPort  ActionType=then
  cfblk3 : simulink/Discrete/Transfer Fcn First Order  PoleZ=0.95  ICPrevOutput=0.0  DoSatur=off
      settings: SourceProductName=Simulink
  cfblk4 : Sum  Inputs=|++
  cfblk5 : Subsystem
  cfblk6 : Subsystem
  cfblk7 : Subsystem
  cfblk8 : Delay
  cfblk2 : Outport
  wires:
  cfblk6/1(cfblk2) -> cfblk7/1(cfblk1), cfblk5/1(cfblk1)
  cfblk1/1 -> cfblk2/1
  cfblk7/1(cfblk2) -> cfblk4/1
  cfblk5/1(cfblk2) -> cfblk4/2
  cfblk3/1 -> cfblk6/1(cfblk1)
  cfblk4/1 -> cfblk8/1
  cfblk8/1 -> cfblk3/1

== system sampleModel111/cfblk150 ==
  cfblk1 : Inport
  cfblk6 : Inport  Port=2
  cfblk7 : Inport  Port=3
  Action Port : ActionPort  ActionType=else
  cfblk10 : Subsystem  TreatAsAtomicUnit=on
  cfblk11 : Delay
  cfblk3 : Sqrt  SaturateOnIntegerOverflow=on
  cfblk4 : Constant  Value=[858281936.424164]  SampleTime=1
  cfblk5 : If  IfExpression=u1 >= 0  SampleTime=1
  cfblk9 : Subsystem  TreatAsAtomicUnit=on
  cfblk2 : Outport
  cfblk8 : Outport  Port=2
  wires:
  cfblk6/1 -> cfblk8/1
  cfblk1/1 -> cfblk10/1(cfblk1)
  cfblk4/1 -> cfblk5/1
  cfblk3/1 -> cfblk9/1(cfblk1)
  cfblk10/1(cfblk2) -> cfblk2/1
  cfblk5/1 -> cfblk9/Action
  cfblk5/2 -> cfblk10/Action
  cfblk9/1(cfblk2) -> cfblk11/1
  cfblk11/1 -> cfblk3/1

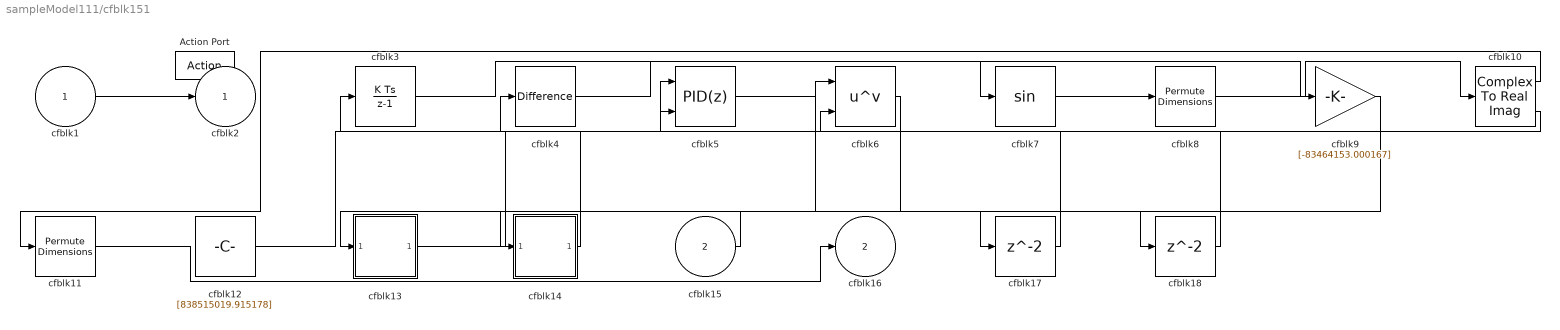
== system sampleModel111/cfblk151 ==
  cfblk1 : Inport
  cfblk15 : Inport  Port=2
  Action Port : ActionPort  ActionType=then
  cfblk10 : ComplexToRealImag
  cfblk11 : PermuteDimensions
  cfblk12 : Constant  Value=[838515019.915178]  SampleTime=1
  cfblk13 : Subsystem
  cfblk14 : Subsystem
  cfblk17 : Delay
  cfblk18 : Delay
  cfblk3 : DiscreteIntegrator  SampleTime=-1  ICPrevOutput=DiscIntNeverNeededParam  ICPrevScaledInput=DiscIntNeverNeededParam
  cfblk4 : simulink/Discrete/Difference  ICPrevInput=0.0  OutMin=[]  OutMax=[]  OutDataTypeStr=Inherit: Inherit via back propagation  OutDataType=fixdt(1, 16)  OutScaling=2^-10  DoSatur=off
  cfblk5 : simulink/Continuous/PID Controller (2DOF)  Controller=PID  TimeDomain=Discrete-time  SampleTime=-1  IntegratorMethod=Forward Euler  FilterMethod=Forward Euler  Form=Parallel  UseFilter=on  ControllerParametersSource=internal  P=1  I=1  D=0  N=100  b=1  c=1  InitialConditionSource=internal  InitialConditionForIntegrator=0  InitialConditionForFilter=0  ExternalReset=none  LimitOutput=off  UpperSaturationLimit=inf  LowerSaturationLimit=-inf  LinearizeAsGain=off  AntiWindupMode=none  Kb=1  TrackingMode=off  Kt=1  PParamMin=[]  PParamMax=[]  IParamMin=[]  IParamMax=[]  DParamMin=[]  DParamMax=[]  NParamMin=[]  NParamMax=[]  bParamMin=[]  bParamMax=[]  cParamMin=[]  cParamMax=[]  KbParamMin=[]  KbParamMax=[]  KtParamMin=[]  KtParamMax=[]  POutMin=[]  POutMax=[]  IOutMin=[]  IOutMax=[]  DOutMin=[]  DOutMax=[]  NOutMin=[]  NOutMax=[]  bOutMin=[]  bOutMax=[]  cOutMin=[]  cOutMax=[]  KbOutMin=[]  KbOutMax=[]  KtOutMin=[]  KtOutMax=[]  IntegratorOutMin=[]  IntegratorOutMax=[]  FilterOutMin=[]  FilterOutMax=[]  SumOutMin=[]  SumOutMax=[]  Sum1OutMin=[]  Sum1OutMax=[]  Sum2OutMin=[]  Sum2OutMax=[]  Sum3OutMin=[]  Sum3OutMax=[]  SumI1OutMin=[]  SumI1OutMax=[]  SumI2OutMin=[]  SumI2OutMax=[]  SumI3OutMin=[]  SumI3OutMax=[]  SumDOutMin=[]  SumDOutMax=[]  SaturationOutMin=[]  SaturationOutMax=[]  IntegratorContinuousStateAttributes=''  IntegratorStateMustResolveToSignalObject=off  IntegratorRTWStateStorageClass=Auto  FilterContinuousStateAttributes=''  FilterStateMustResolveToSignalObject=off  FilterRTWStateStorageClass=Auto  DifferentiatorICPrevScaledInput=0  DifferentiatorOutMin=[]  DifferentiatorOutMax=[]  FilterDiffOutCoefMin=[]  FilterDiffOutCoefMax=[]  SumDenOutMin=[]  SumDenOutMax=[]  SumNumOutMin=[]  SumNumOutMax=[]  ReciprocalOutMin=[]  ReciprocalOutMax=[]  DivideOutMin=[]  DivideOutMax=[]  TunerSelectOption=Transfer Function Based (PID Tuner App)
  cfblk6 : Math  Operator=pow  SaturateOnIntegerOverflow=on
  cfblk7 : Trigonometry
  cfblk8 : PermuteDimensions
  cfblk9 : Gain  Gain=[-83464153.000167]
  cfblk2 : Outport
  cfblk16 : Outport  Port=2
  wires:
  cfblk1/1 -> cfblk2/1
  cfblk8/1 -> cfblk10/1
  cfblk13/1(cfblk2) -> cfblk5/1
  cfblk4/1 -> cfblk7/1
  cfblk7/1 -> cfblk8/1
  cfblk11/1 -> cfblk16/1
  cfblk6/1 -> cfblk13/1(cfblk1)
  cfblk14/1(cfblk2) -> cfblk4/1
  cfblk12/1 -> cfblk5/2
  cfblk15/1 -> cfblk14/1(cfblk1)
  cfblk10/1 -> cfblk11/1
  cfblk10/2 -> cfblk6/2
  cfblk3/1 -> cfblk9/1
  cfblk9/1 -> cfblk17/1
  cfblk17/1 -> cfblk3/1
  cfblk5/1 -> cfblk18/1
  cfblk18/1 -> cfblk6/1

== system sampleModel111/cfblk152 ==
  cfblk1 : Inport
  Action Port : ActionPort  ActionType=else
  cfblk3 : DotProduct  InputSameDT=on  OutDataTypeStr=Inherit: Inherit via internal rule
  cfblk4 : Constant  Value=[940889131.807750]  SampleTime=1
  cfblk5 : Subsystem
  cfblk6 : Subsystem
  cfblk7 : Subsystem
  cfblk8 : Subsystem
  cfblk9 : Subsystem
  cfblk2 : Outport
  cfblk10 : Outport  Port=2
  wires:
  cfblk9/1(cfblk2) -> cfblk10/1
  cfblk1/1 -> cfblk7/1(cfblk1), cfblk3/2
  cfblk5/1(cfblk2) -> cfblk6/1(cfblk1)
  cfblk4/1 -> cfblk3/1
  cfblk8/1(cfblk2) -> cfblk9/1(cfblk1)
  cfblk3/1 -> cfblk5/1(cfblk1)
  cfblk6/1(cfblk2) -> cfblk2/1
  cfblk7/1(cfblk2) -> cfblk8/1(cfblk1)

== system sampleModel111/cfblk153 ==
  cfblk1 : Inport
  cfblk10 : Inport  Port=2
  cfblk11 : Inport  Port=3
  Action Port : ActionPort  ActionType=then
  cfblk14 : Delay
  cfblk15 : Delay
  cfblk3 : MinMax  Function=max  Inputs=2
  cfblk4 : Subsystem
  cfblk5 : Subsystem
  cfblk6 : Subsystem
  cfblk7 : Subsystem
  cfblk8 : Subsystem
  cfblk9 : Subsystem
  cfblk2 : Outport
  cfblk12 : Outport  Port=2
  cfblk13 : Outport  Port=3
  wires:
  cfblk6/1(cfblk2) -> cfblk9/1(cfblk1)
  cfblk9/1(cfblk2) -> cfblk12/1
  cfblk3/1 -> cfblk5/1(cfblk1)
  cfblk7/1(cfblk2) -> cfblk8/1(cfblk1)
  cfblk10/1 -> cfblk13/1
  cfblk11/1 -> cfblk6/1(cfblk1)
  cfblk1/1 -> cfblk2/1
  cfblk8/1(cfblk2) -> cfblk4/1(cfblk1), cfblk15/1
  cfblk4/1(cfblk2) -> cfblk3/1
  cfblk5/1(cfblk2) -> cfblk14/1
  cfblk14/1 -> cfblk3/2
  cfblk15/1 -> cfblk7/1(cfblk1)

== system sampleModel111/cfblk154 ==
  cfblk1 : Inport
  cfblk8 : Inport  Port=2
  cfblk9 : Inport  Port=3
  Action Port : ActionPort  ActionType=else
  cfblk3 : simulink/Discrete/Transfer Fcn First Order  PoleZ=0.95  ICPrevOutput=0.0  DoSatur=off
      settings: SourceProductName=Simulink
  cfblk4 : DiscreteFilter
  cfblk5 : DiscreteTransferFcn
  cfblk6 : Math  Operator=hypot  SaturateOnIntegerOverflow=on
  cfblk7 : Subsystem
  cfblk2 : Outport
  cfblk10 : Outport  Port=2
  wires:
  cfblk7/1(cfblk2) -> cfblk3/1
  cfblk8/1 -> cfblk6/1
  cfblk4/1 -> cfblk6/2
  cfblk9/1 -> cfblk2/1
  cfblk1/1 -> cfblk5/1
  cfblk6/1 -> cfblk10/1
  cfblk5/1 -> cfblk7/1(cfblk1)
  cfblk3/1 -> cfblk4/1

== system sampleModel111/cfblk155 ==
  cfblk1 : Inport
  Action Port : ActionPort  ActionType=then
  cfblk10 : Delay
  cfblk3 : UnitDelay  SampleTime=-1
  cfblk4 : UnitDelay  SampleTime=-1
  cfblk5 : Rounding
  cfblk6 : Constant  Value=[544923772.144001]  SampleTime=1
  cfblk7 : Subsystem
  cfblk8 : Subsystem
  cfblk9 : Subsystem
  cfblk2 : Outport
  wires:
  cfblk5/1 -> cfblk7/1(cfblk1)
  cfblk1/1 -> cfblk4/1
  cfblk9/1(cfblk2) -> cfblk2/1
  cfblk4/1 -> cfblk9/1(cfblk1)
  cfblk6/1 -> cfblk8/1(cfblk1)
  cfblk8/1(cfblk2) -> cfblk3/1
  cfblk7/1(cfblk2) -> cfblk10/1
  cfblk10/1 -> cfblk5/1

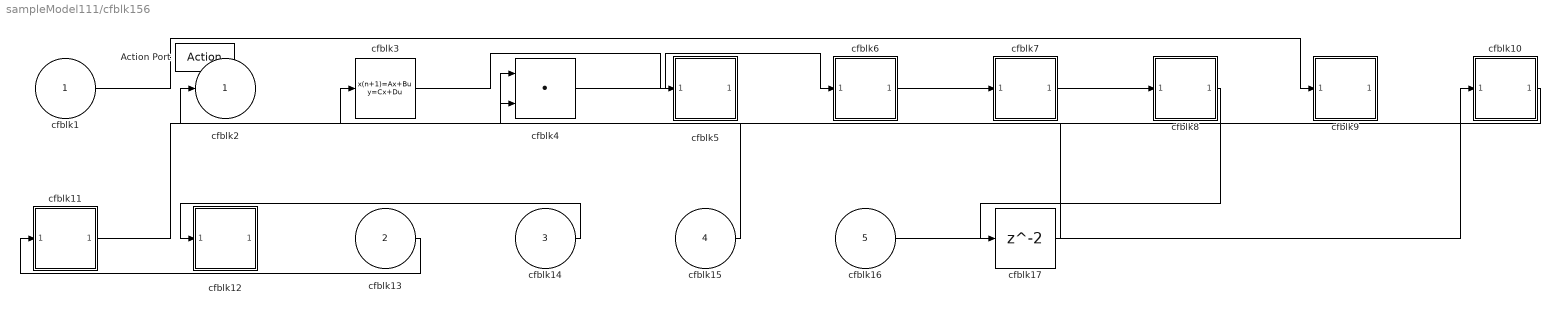
== system sampleModel111/cfblk156 ==
  cfblk1 : Inport
  cfblk13 : Inport  Port=2
  cfblk14 : Inport  Port=3
  cfblk15 : Inport  Port=4
  cfblk16 : Inport  Port=5
  Action Port : ActionPort  ActionType=else
  cfblk10 : Subsystem
  cfblk11 : Subsystem
  cfblk12 : Subsystem
  cfblk17 : Delay
  cfblk3 : DiscreteStateSpace  SampleTime=-1
  cfblk4 : DotProduct  InputSameDT=on  OutDataTypeStr=Inherit: Inherit via internal rule
  cfblk5 : Subsystem
  cfblk6 : Subsystem
  cfblk7 : Subsystem
  cfblk8 : Subsystem
  cfblk9 : Subsystem
  cfblk2 : Outport
  wires:
  cfblk4/1 -> cfblk6/1(cfblk1)
  cfblk14/1 -> cfblk12/1(cfblk1)
  cfblk11/1(cfblk2) -> cfblk3/1
  cfblk1/1 -> cfblk9/1(cfblk1)
  cfblk10/1(cfblk2) -> cfblk4/1
  cfblk15/1 -> cfblk2/1
  cfblk16/1 -> cfblk10/1(cfblk1)
  cfblk7/1(cfblk2) -> cfblk8/1(cfblk1)
  cfblk3/1 -> cfblk5/1(cfblk1)
  cfblk13/1 -> cfblk11/1(cfblk1)
  cfblk6/1(cfblk2) -> cfblk7/1(cfblk1)
  cfblk8/1(cfblk2) -> cfblk17/1
  cfblk17/1 -> cfblk4/2

== system sampleModel111/cfblk157 ==
  cfblk1 : Inport
  cfblk9 : Inport  Port=2
  Action Port : ActionPort  ActionType=then
  cfblk3 : Product  Inputs=**
  cfblk4 : Abs
  cfblk5 : Assignment  DiagnosticForDimensions=Warning  IndexOptions=Index vector (dialog)  Indices=1  OutputSizes=1
  cfblk6 : Constant  Value=[-470385504.632421]  SampleTime=1
  cfblk7 : Subsystem
  cfblk8 : Subsystem
  cfblk2 : Outport
  wires:
  cfblk9/1 -> cfblk8/1(cfblk1)
  cfblk6/1 -> cfblk7/1(cfblk1)
  cfblk1/1 -> cfblk5/1
  cfblk8/1(cfblk2) -> cfblk3/1
  cfblk3/1 -> cfblk5/2
  cfblk4/1 -> cfblk3/2
  cfblk7/1(cfblk2) -> cfblk4/1
  cfblk5/1 -> cfblk2/1

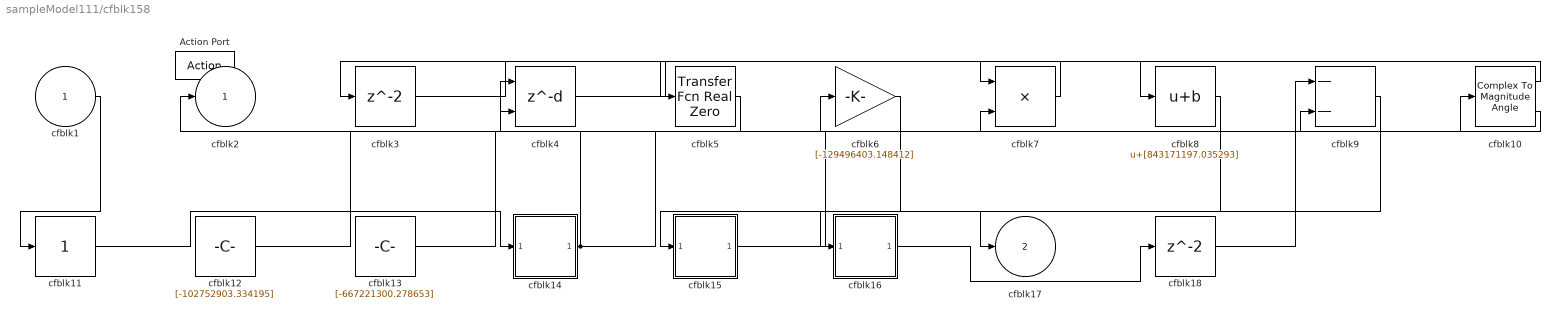
== system sampleModel111/cfblk158 ==
  cfblk1 : Inport
  Action Port : ActionPort  ActionType=else
  cfblk10 : ComplexToMagnitudeAngle
  cfblk11 : simulink/Math Operations/Slider Gain  gain=1  low=0  high=2
  cfblk12 : Constant  Value=[-102752903.334195]  SampleTime=1
  cfblk13 : Constant  Value=[-667221300.278653]  SampleTime=1
  cfblk14 : Subsystem
  cfblk15 : Subsystem
  cfblk16 : Subsystem
  cfblk18 : Delay
  cfblk3 : Delay
  cfblk4 : Delay  DelayLengthSource=Input port
      settings: InputPortMap=u0,p1
  cfblk5 : simulink/Discrete/Transfer Fcn Real Zero  ZeroZ=0.75  ICPrevInput=0.0  DoSatur=off
      settings: SourceProductName=Simulink  SourceProductBaseCode=SL
  cfblk6 : Gain  Gain=[-129496403.148412]
  cfblk7 : Product
  cfblk8 : Bias  Bias=[843171197.035293]
  cfblk9 : Sum  Inputs=--
  cfblk2 : Outport
  cfblk17 : Outport  Port=2
  wires:
  cfblk5/1 -> cfblk2/1
  cfblk15/1(cfblk2) -> cfblk10/1
  cfblk4/1 -> cfblk8/1
  cfblk6/1 -> cfblk15/1(cfblk1)
  cfblk10/1 -> cfblk7/1
  cfblk14/1(cfblk2) -> cfblk9/2, cfblk4/2
  cfblk3/1 -> cfblk5/1
  cfblk9/1 -> cfblk16/1(cfblk1)
  cfblk8/1 -> cfblk17/1
  cfblk1/1 -> cfblk11/1
  cfblk11/1 -> cfblk14/1(cfblk1)
  cfblk7/1 -> cfblk3/1
  cfblk13/1 -> cfblk7/2
  cfblk10/2 -> cfblk4/1
  cfblk12/1 -> cfblk6/1
  cfblk16/1(cfblk2) -> cfblk18/1
  cfblk18/1 -> cfblk9/1

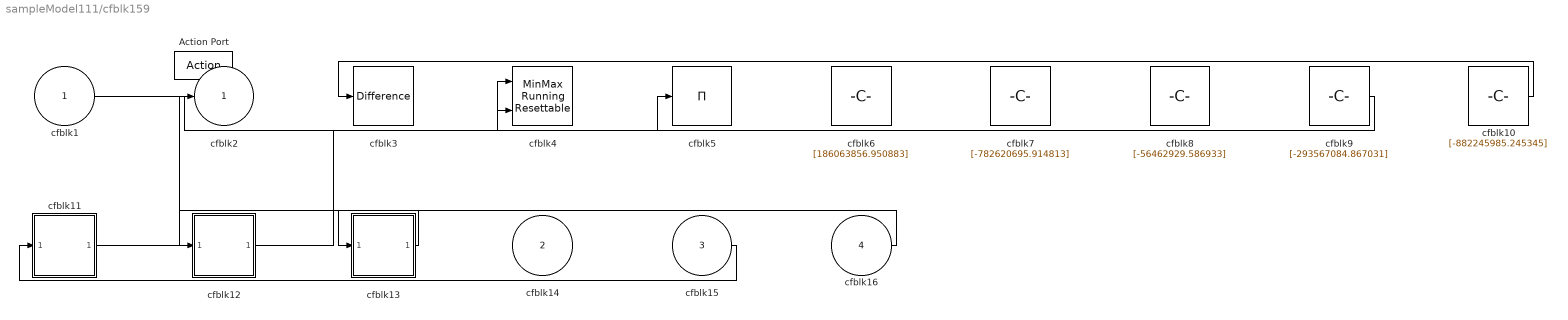
== system sampleModel111/cfblk159 ==
  cfblk1 : Inport
  cfblk14 : Inport  Port=2
  cfblk15 : Inport  Port=3
  cfblk16 : Inport  Port=4
  Action Port : ActionPort  ActionType=then
  cfblk10 : Constant  Value=[-882245985.245345]  SampleTime=1
  cfblk11 : Subsystem
  cfblk12 : Subsystem
  cfblk13 : Subsystem
  cfblk3 : simulink/Discrete/Difference  ICPrevInput=0.0  OutMin=[]  OutMax=[]  OutDataTypeStr=Inherit: Inherit via back propagation  OutDataType=fixdt(1, 16)  OutScaling=2^-10  DoSatur=off
  cfblk4 : simulink/Math Operations/MinMax Running Resettable  Function=min  vinit=0.0
  cfblk5 : Product  Inputs=*
  cfblk6 : Constant  Value=[186063856.950883]  SampleTime=1
  cfblk7 : Constant  Value=[-782620695.914813]  SampleTime=1
  cfblk8 : Constant  Value=[-56462929.586933]  SampleTime=1
  cfblk9 : Constant  Value=[-293567084.867031]  SampleTime=1
  cfblk2 : Outport
  wires:
  cfblk1/1 -> cfblk5/1
  cfblk11/1(cfblk2) -> cfblk2/1
  cfblk15/1 -> cfblk11/1(cfblk1)
  cfblk13/1(cfblk2) -> cfblk12/1(cfblk1)
  cfblk16/1 -> cfblk13/1(cfblk1)
  cfblk10/1 -> cfblk3/1
  cfblk12/1(cfblk2) -> cfblk4/1
  cfblk9/1 -> cfblk4/2

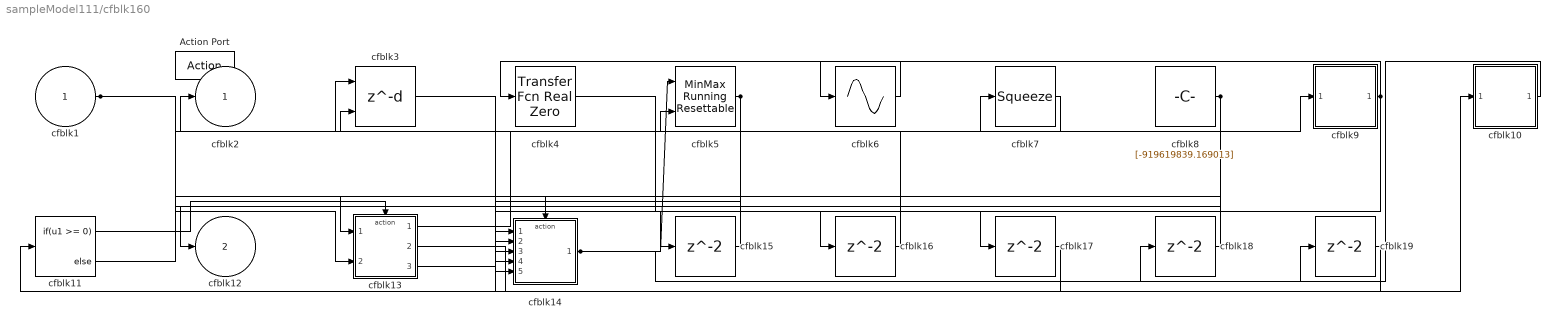
== system sampleModel111/cfblk160 ==
  cfblk1 : Inport
  Action Port : ActionPort  ActionType=else
  cfblk10 : Subsystem
  cfblk11 : If  IfExpression=u1 >= 0  SampleTime=1
  cfblk13 : Subsystem  TreatAsAtomicUnit=on
  cfblk14 : Subsystem  TreatAsAtomicUnit=on
  cfblk{15..19} (5 alike) : Delay
  cfblk3 : Delay  DelayLengthSource=Input port
      settings: InputPortMap=u0,p1
  cfblk4 : simulink/Discrete/Transfer Fcn Real Zero  ZeroZ=0.75  ICPrevInput=0.0  DoSatur=off
      settings: SourceProductName=Simulink  SourceProductBaseCode=SL
  cfblk5 : simulink/Math Operations/MinMax Running Resettable  Function=min  vinit=0.0
  cfblk6 : Sin  TimeSource=Use external signal  SampleTime=0
  cfblk7 : Squeeze
  cfblk8 : Constant  Value=[-919619839.169013]  SampleTime=1
  cfblk9 : Subsystem
  cfblk2 : Outport
  cfblk12 : Outport  Port=2
  wires:
  cfblk13/1(cfblk2) -> cfblk9/1(cfblk1)
  cfblk9/1(cfblk2) -> cfblk6/1, cfblk17/1
  cfblk6/1 -> cfblk4/1
  cfblk13/2(cfblk16) -> cfblk10/1(cfblk1)
  cfblk3/1 -> cfblk14/1(cfblk1)
  cfblk5/1 -> cfblk2/1, cfblk15/1
  cfblk14/1(cfblk2) -> cfblk5/1, cfblk19/1
  cfblk13/3(cfblk17) -> cfblk7/1
  cfblk1/1 -> cfblk3/2, cfblk13/2(cfblk15), cfblk14/4(cfblk14)
  cfblk8/1 -> cfblk12/1, cfblk14/5(cfblk15)
  cfblk7/1 -> cfblk5/2
  cfblk11/1 -> cfblk13/Action
  cfblk11/2 -> cfblk14/Action
  cfblk15/1 -> cfblk14/2(cfblk12)
  cfblk4/1 -> cfblk16/1
  cfblk16/1 -> cfblk3/1
  cfblk17/1 -> cfblk14/3(cfblk13)
  cfblk10/1(cfblk2) -> cfblk18/1
  cfblk18/1 -> cfblk13/1(cfblk1)
  cfblk19/1 -> cfblk11/1

== system sampleModel111/cfblk161 ==
  cfblk1 : Inport
  Action Port : ActionPort  ActionType=then
  cfblk3 : DiscreteFir
  cfblk4 : Squeeze
  cfblk5 : UnaryMinus
  cfblk6 : Subsystem
  cfblk7 : Subsystem
  cfblk2 : Outport
  wires:
  cfblk3/1 -> cfblk7/1(cfblk1)
  cfblk1/1 -> cfblk5/1
  cfblk6/1(cfblk2) -> cfblk3/1
  cfblk7/1(cfblk2) -> cfblk4/1
  cfblk5/1 -> cfblk6/1(cfblk1)
  cfblk4/1 -> cfblk2/1

== system sampleModel111/cfblk162 ==
  cfblk1 : Inport
  cfblk7 : Inport  Port=2
  Action Port : ActionPort  ActionType=else
  cfblk3 : simulink/Math Operations/MinMax Running Resettable  Function=min  vinit=0.0
  cfblk4 : Sum  Inputs=|++
  cfblk5 : Constant  Value=[297950737.938677]  SampleTime=1
  cfblk6 : Subsystem
  cfblk8 : Delay
  cfblk2 : Outport
  wires:
  cfblk3/1 -> cfblk4/1
  cfblk1/1 -> cfblk6/1(cfblk1)
  cfblk7/1 -> cfblk2/1
  cfblk5/1 -> cfblk4/2
  cfblk6/1(cfblk2) -> cfblk3/2
  cfblk4/1 -> cfblk8/1
  cfblk8/1 -> cfblk3/1

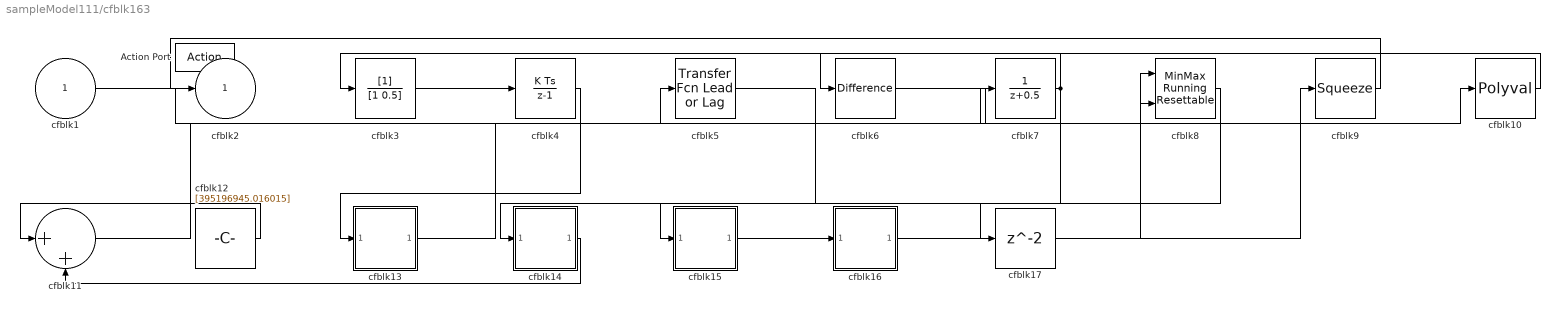
== system sampleModel111/cfblk163 ==
  cfblk1 : Inport
  Action Port : ActionPort  ActionType=then
  cfblk10 : Polyval  Coefs=[ +2.081618890e-019, -1.441693666e-014, +4.719686976e-010, -8.536869453e-006, +1.621573104e-001, -8.087801117e+001 ]
  cfblk11 : Sum  Inputs=|++
  cfblk12 : Constant  Value=[395196945.016015]  SampleTime=1
  cfblk13 : Subsystem
  cfblk14 : Subsystem
  cfblk15 : Subsystem
  cfblk16 : Subsystem
  cfblk17 : Delay
  cfblk3 : DiscreteFilter
  cfblk4 : DiscreteIntegrator  SampleTime=-1  ICPrevOutput=DiscIntNeverNeededParam  ICPrevScaledInput=DiscIntNeverNeededParam
  cfblk5 : simulink/Discrete/Transfer Fcn Lead or Lag  PoleZ=0.95  ZeroZ=0.75  ICPrevOutput=0.0  ICPrevInput=0.0  DoSatur=off
      settings: SourceProductName=Simulink  SourceProductBaseCode=SL
  cfblk6 : simulink/Discrete/Difference  ICPrevInput=0.0  OutMin=[]  OutMax=[]  OutDataTypeStr=Inherit: Inherit via back propagation  OutDataType=fixdt(1, 16)  OutScaling=2^-10  DoSatur=off
  cfblk7 : DiscreteTransferFcn
  cfblk8 : simulink/Math Operations/MinMax Running Resettable  Function=min  vinit=0.0
  cfblk9 : Squeeze
  cfblk2 : Outport
  wires:
  cfblk15/1(cfblk2) -> cfblk16/1(cfblk1)
  cfblk8/1 -> cfblk14/1(cfblk1)
  cfblk9/1 -> cfblk2/1
  cfblk7/1 -> cfblk3/1, cfblk15/1(cfblk1)
  cfblk6/1 -> cfblk8/1
  cfblk4/1 -> cfblk13/1(cfblk1)
  cfblk16/1(cfblk2) -> cfblk9/1
  cfblk1/1 -> cfblk7/1
  cfblk12/1 -> cfblk11/1
  cfblk3/1 -> cfblk4/1
  cfblk10/1 -> cfblk6/1
  cfblk14/1(cfblk2) -> cfblk11/2
  cfblk13/1(cfblk2) -> cfblk10/1
  cfblk11/1 -> cfblk5/1
  cfblk5/1 -> cfblk17/1
  cfblk17/1 -> cfblk8/2

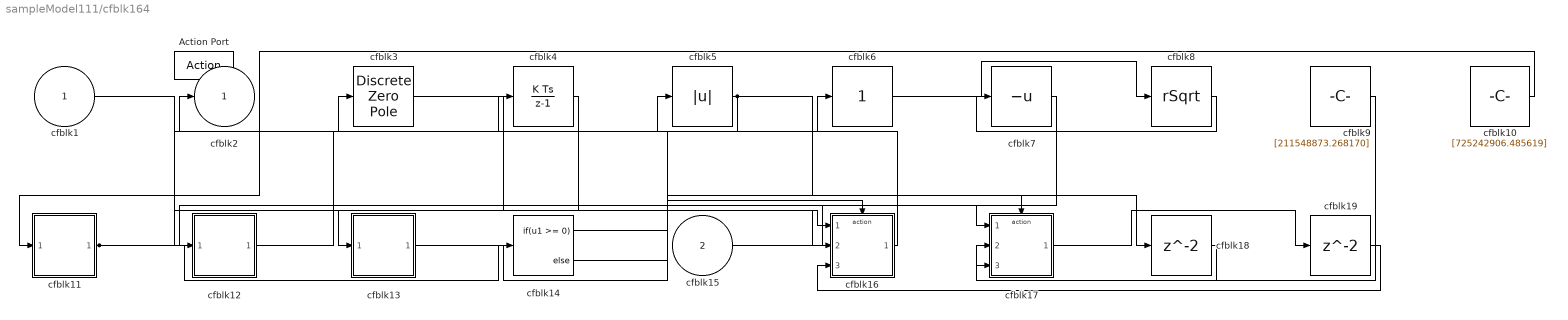
== system sampleModel111/cfblk164 ==
  cfblk1 : Inport
  cfblk15 : Inport  Port=2
  Action Port : ActionPort  ActionType=else
  cfblk10 : Constant  Value=[725242906.485619]  SampleTime=1
  cfblk11 : Subsystem
  cfblk12 : Subsystem
  cfblk13 : Subsystem
  cfblk14 : If  IfExpression=u1 >= 0  SampleTime=1
  cfblk16 : Subsystem  TreatAsAtomicUnit=on
  cfblk17 : Subsystem  TreatAsAtomicUnit=on
  cfblk18 : Delay
  cfblk19 : Delay
  cfblk3 : DiscreteZeroPole  Poles=[0 0.5]  Gain=1  SampleTime=-1
  cfblk4 : DiscreteIntegrator  SampleTime=-1  ICPrevOutput=DiscIntNeverNeededParam  ICPrevScaledInput=DiscIntNeverNeededParam
  cfblk5 : Abs
  cfblk6 : simulink/Math Operations/Slider Gain  gain=1  low=0  high=2
  cfblk7 : UnaryMinus
  cfblk8 : Sqrt  Operator=rSqrt  AlgorithmType=Newton-Raphson  SaturateOnIntegerOverflow=on
  cfblk9 : Constant  Value=[211548873.268170]  SampleTime=1
  cfblk2 : Outport
  wires:
  cfblk6/1 -> cfblk8/1
  cfblk4/1 -> cfblk13/1(cfblk1)
  cfblk15/1 -> cfblk17/1(cfblk1)
  cfblk13/1(cfblk2) -> cfblk6/1
  cfblk8/1 -> cfblk7/1
  cfblk11/1(cfblk2) -> cfblk14/1, cfblk3/1
  cfblk7/1 -> cfblk12/1(cfblk1)
  cfblk3/1 -> cfblk16/1(cfblk1)
  cfblk10/1 -> cfblk11/1(cfblk1)
  cfblk16/1(cfblk2) -> cfblk4/1
  cfblk12/1(cfblk2) -> cfblk5/1
  cfblk9/1 -> cfblk17/2(cfblk13)
  cfblk5/1 -> cfblk2/1, cfblk18/1
  cfblk1/1 -> cfblk16/2(cfblk7)
  cfblk14/1 -> cfblk16/Action
  cfblk14/2 -> cfblk17/Action
  cfblk18/1 -> cfblk17/3(cfblk14)
  cfblk17/1(cfblk2) -> cfblk19/1
  cfblk19/1 -> cfblk16/3(cfblk8)

== system sampleModel111/cfblk165 ==
  cfblk1 : Inport
  cfblk10 : Inport  Port=2
  cfblk11 : Inport  Port=3
  Action Port : ActionPort  ActionType=then
  cfblk3 : simulink/Continuous/PID Controller (2DOF)  Controller=PID  TimeDomain=Discrete-time  SampleTime=-1  IntegratorMethod=Forward Euler  FilterMethod=Forward Euler  Form=Parallel  UseFilter=on  ControllerParametersSource=internal  P=1  I=1  D=0  N=100  b=1  c=1  InitialConditionSource=internal  InitialConditionForIntegrator=0  InitialConditionForFilter=0  ExternalReset=none  LimitOutput=off  UpperSaturationLimit=inf  LowerSaturationLimit=-inf  LinearizeAsGain=off  AntiWindupMode=none  Kb=1  TrackingMode=off  Kt=1  PParamMin=[]  PParamMax=[]  IParamMin=[]  IParamMax=[]  DParamMin=[]  DParamMax=[]  NParamMin=[]  NParamMax=[]  bParamMin=[]  bParamMax=[]  cParamMin=[]  cParamMax=[]  KbParamMin=[]  KbParamMax=[]  KtParamMin=[]  KtParamMax=[]  POutMin=[]  POutMax=[]  IOutMin=[]  IOutMax=[]  DOutMin=[]  DOutMax=[]  NOutMin=[]  NOutMax=[]  bOutMin=[]  bOutMax=[]  cOutMin=[]  cOutMax=[]  KbOutMin=[]  KbOutMax=[]  KtOutMin=[]  KtOutMax=[]  IntegratorOutMin=[]  IntegratorOutMax=[]  FilterOutMin=[]  FilterOutMax=[]  SumOutMin=[]  SumOutMax=[]  Sum1OutMin=[]  Sum1OutMax=[]  Sum2OutMin=[]  Sum2OutMax=[]  Sum3OutMin=[]  Sum3OutMax=[]  SumI1OutMin=[]  SumI1OutMax=[]  SumI2OutMin=[]  SumI2OutMax=[]  SumI3OutMin=[]  SumI3OutMax=[]  SumDOutMin=[]  SumDOutMax=[]  SaturationOutMin=[]  SaturationOutMax=[]  IntegratorContinuousStateAttributes=''  IntegratorStateMustResolveToSignalObject=off  IntegratorRTWStateStorageClass=Auto  FilterContinuousStateAttributes=''  FilterStateMustResolveToSignalObject=off  FilterRTWStateStorageClass=Auto  DifferentiatorICPrevScaledInput=0  DifferentiatorOutMin=[]  DifferentiatorOutMax=[]  FilterDiffOutCoefMin=[]  FilterDiffOutCoefMax=[]  SumDenOutMin=[]  SumDenOutMax=[]  SumNumOutMin=[]  SumNumOutMax=[]  ReciprocalOutMin=[]  ReciprocalOutMax=[]  DivideOutMin=[]  DivideOutMax=[]  TunerSelectOption=Transfer Function Based (PID Tuner App)
  cfblk4 : simulink/Discrete/Transfer Fcn Real Zero  ZeroZ=0.75  ICPrevInput=0.0  DoSatur=off
      settings: SourceProductName=Simulink  SourceProductBaseCode=SL
  cfblk5 : Delay  ShowEnablePort=on
      settings: InputPortMap=u0,e6
  cfblk6 : PermuteDimensions
  cfblk7 : Signum
  cfblk8 : Constant  Value=[-604109303.066319]  SampleTime=1
  cfblk9 : Subsystem
  cfblk2 : Outport
  wires:
  cfblk7/1 -> cfblk6/1
  cfblk9/1(cfblk2) -> cfblk7/1
  cfblk11/1 -> cfblk4/1
  cfblk6/1 -> cfblk5/1
  cfblk4/1 -> cfblk5/2
  cfblk10/1 -> cfblk9/1(cfblk1)
  cfblk8/1 -> cfblk2/1
  cfblk1/1 -> cfblk3/1
  cfblk5/1 -> cfblk3/2
